simulink model "testpend"  (R2024b)
settings: Solver=VariableStepAuto  StartTime=0.0  StopTime=10  RelTol=1e-3
values from neighbouring files (symbols this model uses):
  A = [0   1.0000        0        0 ... (first row only)    [invgui.m]    (also in p1.m = 14; p2.m = 14; robot.m = [0 1 0 0; robot_cascade.m = [ 0, 1, 0, 0)
  B = [0; 1.8182; 0; 4.5455]    [invgui.m]    (also in p1.m = 18; p2.m = 18; robot.m = B ./ R; robot_cascade.m = B ./ r_wheel)
  Cx = C(1,:)    [robot.m]    (also in robot_cascade.m; robot_linear.m; robot_lqr.m)
  x0 = [0 0 0 0]    [invgui.m]    (also in robot.m = [0; 0; 5*pi/180; 0]; robot_cascade.m = [0; 0; 5*pi/180; 0]; robot_linear.m = [0; 0; 5*pi/180; 0]; robot_lqr.m = [0; 0; 5*pi/180; 0])
undefined symbols (not defined in the file or in its folder): Ad, Bd, Cd, K_d, Ob
settings Model: Creator=cosr3  LastModifiedBy=cosr3

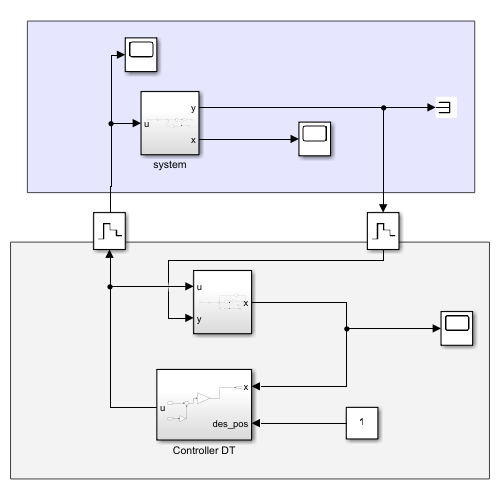
[thumbnail: Simulink's stored preview of the top-level diagram]
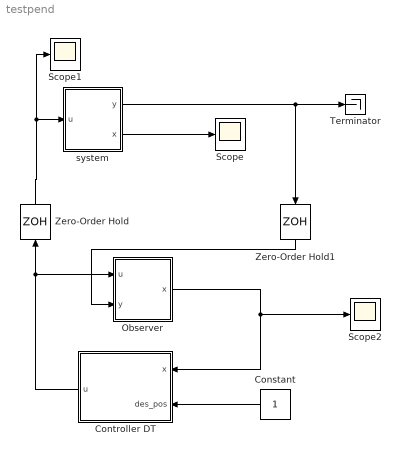
== system testpend ==
  Constant : Constant
  Controller DT : Subsystem
  Observer : Subsystem
  Scope : Scope
  Scope1 : Scope
  Scope2 : Scope
  Terminator : Terminator
  Zero-Order Hold : ZeroOrderHold  SampleTime=-1
  Zero-Order Hold1 : ZeroOrderHold  SampleTime=-1
  system : Subsystem
  wires:
  system/1(y) -> Zero-Order Hold1/1, Terminator/1
  system/2(x) -> Scope/1
  Controller DT/1(u) -> Observer/1(u), Zero-Order Hold/1
  Constant/1 -> Controller DT/2(des_pos)
  Zero-Order Hold/1 -> Scope1/1, system/1(u)
  Zero-Order Hold1/1 -> Observer/2(y)
  Observer/1(x) -> Controller DT/1(x), Scope2/1

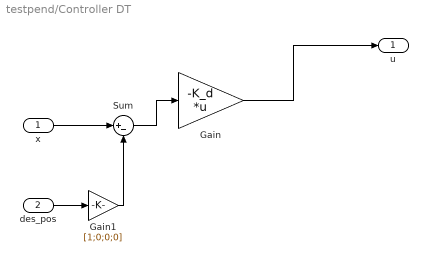
== system testpend/Controller DT ==
  x : Inport
  des_pos : Inport  Port=2
  Gain : Gain  Gain=-K_d  Multiplication=Matrix(K*u) (u vector)
  Gain1 : Gain  Gain=[1;0;0;0]
  Sum : Sum  Inputs=|+-
  u : Outport
  wires:
  Gain/1 -> u/1
  x/1 -> Sum/1
  Sum/1 -> Gain/1
  des_pos/1 -> Gain1/1
  Gain1/1 -> Sum/2

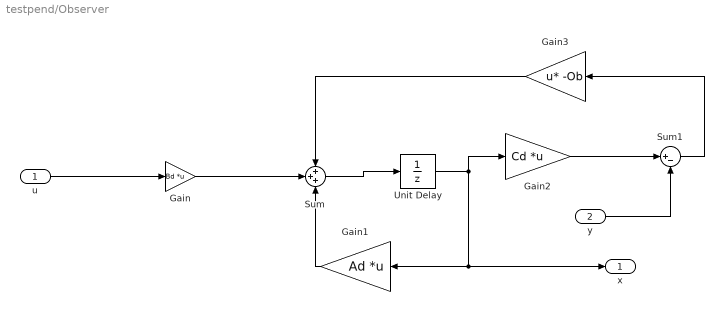
== system testpend/Observer ==
  u : Inport
  y : Inport  Port=2
  Gain : Gain  Gain=Bd  Multiplication=Matrix(K*u)
  Gain1 : Gain  Gain=Ad  Multiplication=Matrix(K*u) (u vector)
  Gain2 : Gain  Gain=Cd  Multiplication=Matrix(K*u)
  Gain3 : Gain  Gain=-Ob  Multiplication=Matrix(u*K)
  Sum : Sum  Inputs=+++
  Sum1 : Sum  Inputs=|+-
  Unit Delay : UnitDelay  InitialCondition=x0*0  SampleTime=-1  HasFrameUpgradeWarning=on
  x : Outport
  wires:
  Sum/1 -> Unit Delay/1
  Gain/1 -> Sum/2
  u/1 -> Gain/1
  Gain1/1 -> Sum/3
  Gain2/1 -> Sum1/1
  Unit Delay/1 -> Gain1/1, x/1, Gain2/1
  y/1 -> Sum1/2
  Sum1/1 -> Gain3/1
  Gain3/1 -> Sum/1

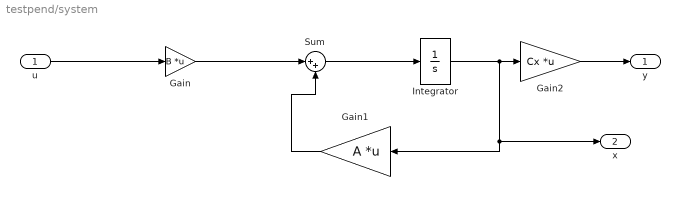
== system testpend/system ==
  u : Inport
  Gain : Gain  Gain=B  Multiplication=Matrix(K*u)
  Gain1 : Gain  Gain=A  Multiplication=Matrix(K*u) (u vector)
  Gain2 : Gain  Gain=Cx  Multiplication=Matrix(K*u) (u vector)
  Integrator : Integrator  InitialCondition=x0
  Sum : Sum  Inputs=|++
  y : Outport
  x : Outport  Port=2
  wires:
  Sum/1 -> Integrator/1
  Gain/1 -> Sum/1
  Integrator/1 -> Gain2/1, x/1, Gain1/1
  u/1 -> Gain/1
  Gain1/1 -> Sum/2
  Gain2/1 -> y/1
